simulink model "kf_discrete_time_1_input"  (R2018b)
settings: Solver=FixedStepAuto  StartTime=0.0  StopTime=15  FixedStep=1e-3  RelTol=1e-3
values from neighbouring files (symbols this model uses):
  A = obj.A    [LeftLaneChangeRelativeMotionModel.m]    (also in initialization.m = 1.75; laneChangeSinusoidalFcn.m = 1.75; laneChangeSinusoidalJacobianFcn.m = 1.75; leftLaneChangeParametricFcn.m = lateral_dist/2)
  Ts = 0.1    [KinematicBicycleModel.m]    (also in LeftLaneChangeSinusoidalMotionModel.m; LinearizedBicycleModel.m; SimplifiedKinematicBicycleModel.m; amm_rel_test.m)
  vx = X(2)    [cv_model_fun.m]    (also in initialization.m = 10)
  vy = X(4)    [cv_model_fun.m]    (also in initialization.m = 0)
  w = obj.w    [LeftLaneChangeRelativeMotionModel.m]    (also in ctra_model_fun.m = X(6); ctrv_model_fun.m = X(5); initialization.m = 0.0314159265359; laneChangeSinusoidalFcn.m = 0.0209439510239)
  x = X(1)    [KinematicBicycleModel.m]    (also in SimplifiedKinematicBicycleModel.m; behavior_model.m = 0:0.01:20; cca_model_fun.m; ctra_model_fun.m)
  y = X(2)    [KinematicBicycleModel.m]    (also in SimplifiedKinematicBicycleModel.m; behavior_model.m = [distances velocities]; cca_model_fun.m; ctra_model_fun.m)
  y_init = lanewidth/2    (= 1.75)    [initialization.m]    (also in laneChangeSinusoidalFcn.m; laneChangeSinusoidalJacobianFcn.m; leftLaneChangeSinusoidalFcn.m; leftLaneChangeSinusoidalJacobianFcn.m)
undefined symbols (not defined in the file or in its folder): Discrete, Time
libraries: simulink x8, sharedTrackingLibrary x2, ctrlSharedLib x1
settings Model: Creator=jasprit  LastModifiedBy=jasprit
settings SFSimCC: SimUseLocalCustomCode=off
settings RTWCC: RTWUseLocalCustomCode=off

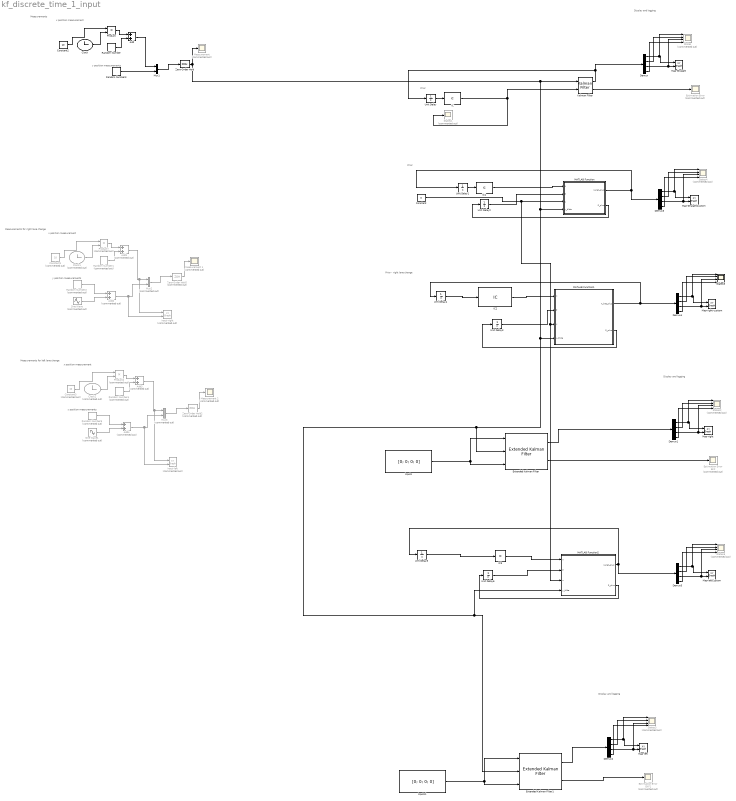
== system kf_discrete_time_1_input ==
  note: Prior - right lane change
  note: Prior
  note: y position measurements
  note: x position measurement
  note: Display and logging
  note: Prior
  note: Measurements
  note: x position measurement
  note: Display and logging
  note: Measurements for right lane change
  note: y position measurements
  note: y position measurements
  note: Measurements for left lane change
  note: Display and logging
  note: x position measurement
  Add : Sum
  Add{1..4} (4 alike) : Sum  Commented=on
  Clock : Clock
  Clock1 : Clock  Commented=on
  Clock2 : Clock  Commented=on
  Constant : Constant  Value=0
  Constant1 : Constant  Commented=on  Value=10
  Constant2 : Constant  Value=10
  Constant3 : Constant  Commented=on  Value=10
  Demux{,1..5} (6 alike) : Demux
  Estimation Error : Scope  Commented=on
  Estimation Error EKF : Scope  Commented=on
  Estimation Error EKF1 : Scope  Commented=on
  Extended Kalman Filter : sharedTrackingLibrary/Extended Kalman Filter  StateTransitionFcn=laneChangeSinusoidalFcn  HasStateTransitionJacobianFcn=on  StateTransitionJacobianFcn=laneChangeSinusoidalJacobianFcn  HasAdditiveProcessNoise=Additive  ProcessNoise=[0.5 5 0.5 5]'  HasTimeVaryingProcessNoise=off  HasStateTransitionFcnExtraArgument=1  InitialState=[x vx y vy]  InitialStateCovariance=1e-6  MeasurementFcn1=positionMeasurementFcn  HasMeasurementJacobianFcn1=off  HasMeasurementEnablePort1=off  HasAdditiveMeasurementNoise1=Additive  MeasurementNoise1=[0.2 0; 0 0.2]  HasTimeVaryingMeasurementNoise1=off  HasMeasurementFcnExtraArgument1=1  MeasurementFcn2=myMeasurementFcn  HasMeasurementJacobianFcn2=off  HasMeasurementEnablePort2=off  HasAdditiveMeasurementNoise2=Additive  MeasurementNoise2=1  HasTimeVaryingMeasurementNoise2=off  HasMeasurementFcnExtraArgument2=0  MeasurementFcn3=myMeasurementFcn  HasMeasurementJacobianFcn3=off  HasMeasurementEnablePort3=off  HasAdditiveMeasurementNoise3=Additive  MeasurementNoise3=1  HasTimeVaryingMeasurementNoise3=off  HasMeasurementFcnExtraArgument3=0  MeasurementFcn4=myMeasurementFcn  HasMeasurementJacobianFcn4=off  HasMeasurementEnablePort4=off  HasAdditiveMeasurementNoise4=Additive  MeasurementNoise4=1  HasTimeVaryingMeasurementNoise4=off  HasMeasurementFcnExtraArgument4=0  MeasurementFcn5=myMeasurementFcn  HasMeasurementJacobianFcn5=off  HasMeasurementEnablePort5=off  HasAdditiveMeasurementNoise5=Additive  MeasurementNoise5=1  HasTimeVaryingMeasurementNoise5=off  HasMeasurementFcnExtraArgument5=0  EnableMultirate=off  StateTransitionFcnSampleTime=1  MeasurementFcn1SampleTime=1  MeasurementFcn2SampleTime=1  MeasurementFcn3SampleTime=1  MeasurementFcn4SampleTime=1  MeasurementFcn5SampleTime=1  UseCurrentEstimator=on  OutputStateCovariance=on  DataType=double  SampleTime=Ts  NumberOfMeasurements=1
      settings: SourceProductName=Control System Toolbox  SourceProductBaseCode=CT
  Extended Kalman Filter1 : sharedTrackingLibrary/Extended Kalman Filter  StateTransitionFcn=leftLaneChangeSinusoidalFcn  HasStateTransitionJacobianFcn=on  StateTransitionJacobianFcn=leftLaneChangeSinusoidalJacobianFcn  HasAdditiveProcessNoise=Additive  ProcessNoise=[0.5 5 0.5 5]'  HasTimeVaryingProcessNoise=off  HasStateTransitionFcnExtraArgument=1  InitialState=[x vx y vy]  InitialStateCovariance=1e-6  MeasurementFcn1=positionMeasurementFcn  HasMeasurementJacobianFcn1=off  HasMeasurementEnablePort1=off  HasAdditiveMeasurementNoise1=Additive  MeasurementNoise1=[0.2 0; 0 0.2]  HasTimeVaryingMeasurementNoise1=off  HasMeasurementFcnExtraArgument1=1  MeasurementFcn2=myMeasurementFcn  HasMeasurementJacobianFcn2=off  HasMeasurementEnablePort2=off  HasAdditiveMeasurementNoise2=Additive  MeasurementNoise2=1  HasTimeVaryingMeasurementNoise2=off  HasMeasurementFcnExtraArgument2=0  MeasurementFcn3=myMeasurementFcn  HasMeasurementJacobianFcn3=off  HasMeasurementEnablePort3=off  HasAdditiveMeasurementNoise3=Additive  MeasurementNoise3=1  HasTimeVaryingMeasurementNoise3=off  HasMeasurementFcnExtraArgument3=0  MeasurementFcn4=myMeasurementFcn  HasMeasurementJacobianFcn4=off  HasMeasurementEnablePort4=off  HasAdditiveMeasurementNoise4=Additive  MeasurementNoise4=1  HasTimeVaryingMeasurementNoise4=off  HasMeasurementFcnExtraArgument4=0  MeasurementFcn5=myMeasurementFcn  HasMeasurementJacobianFcn5=off  HasMeasurementEnablePort5=off  HasAdditiveMeasurementNoise5=Additive  MeasurementNoise5=1  HasTimeVaryingMeasurementNoise5=off  HasMeasurementFcnExtraArgument5=0  EnableMultirate=off  StateTransitionFcnSampleTime=1  MeasurementFcn1SampleTime=1  MeasurementFcn2SampleTime=1  MeasurementFcn3SampleTime=1  MeasurementFcn4SampleTime=1  MeasurementFcn5SampleTime=1  UseCurrentEstimator=on  OutputStateCovariance=on  DataType=double  SampleTime=Ts  NumberOfMeasurements=1
      settings: SourceProductName=Control System Toolbox  SourceProductBaseCode=CT
  IC{,1..3} (4 alike) : InitialCondition  Value=[x vx y vy]
  Inputs : Constant  Value=[0; 0; 0; 0]  SampleTime=Ts
  Inputs1 : Constant  Value=[0; 0; 0; 0]  SampleTime=Ts
  Kalman Filter : ctrlSharedLib/Kalman Filter  TimeDomain=Discrete-Time  UseCurrentEstimator=on  ModelSource=Individual A, B, C, D matrices  ModelSourceVariable=ss(0.95,1,1,0,1)  A=[1 Ts 0 0; 0 1 0 0; 0 0 1 Ts; 0 0 0 1]  B=[1 0; 0 1]  C=[1 0 0 0; 0 0 1 0]  D=[0 0; 0 0]  NumberOfStates=1  NumberOfInputs=1  NumberOfOutputs=1  InitialEstimateSource=Input port  X0=[0 0 20 0]  P0=10  UseK=off  UseGH=off  NumberOfProcessNoiseInputs=1  G=1  TimeInvariantG=on  H=0  TimeInvariantH=on  Q=[0.5 5 0.5 5]'  TimeInvariantQ=on  R=[0.2 0; 0 0.2]  TimeInvariantR=on  N=0  TimeInvariantN=on  AddInputPort=off  AddEnablePort=off  OutputEstimatedY=off  OutputP=on  Ts=Ts
      settings: SourceProductBaseCode=CT
  MATLAB Function : MATLAB Function  TreatAsAtomicUnit=on
  MATLAB Function1 : MATLAB Function  TreatAsAtomicUnit=on
  MATLAB Function2 : MATLAB Function  TreatAsAtomicUnit=on
  Map-Straight : simulink/Sinks/XY Graph  xmin=-1  xmax=200  ymin=-20  ymax=20  st=-1
  Map-StraightCustom : simulink/Sinks/XY Graph  xmin=-1  xmax=200  ymin=-20  ymax=20  st=-1
  Map-left : simulink/Sinks/XY Graph  xmin=-1  xmax=200  ymin=-5  ymax=5  st=-1
  Map-leftCustom : simulink/Sinks/XY Graph  xmin=-1  xmax=200  ymin=-5  ymax=5  st=-1
  Map-right : simulink/Sinks/XY Graph  xmin=-1  xmax=200  ymin=-5  ymax=5  st=-1
  Map-right-custom : simulink/Sinks/XY Graph  xmin=-1  xmax=200  ymin=-5  ymax=5  st=-1
  "Measurement " : Scope  Commented=on
  Measurement 1 : Scope  Commented=on
  Measurement 2 : Scope  Commented=on
  Mux1 : Mux  Inputs=2
  Mux2 : Mux  Commented=on  Inputs=2
  Mux3 : Mux  Commented=on  Inputs=2
  Product : Product
  Product1 : Product  Commented=on
  Product2 : Product  Commented=on
  Random Number : RandomNumber  Variance=0.1  SampleTime=Ts
  Random Number1 : RandomNumber  Commented=on  Variance=0.1  SampleTime=Ts
  Random Number2 : RandomNumber  Commented=on  Variance=0.2  SampleTime=Ts
  Random Number3 : RandomNumber  Variance=0.2  SampleTime=Ts
  Random Number4 : RandomNumber  Commented=on  Variance=0.1  SampleTime=Ts
  Random Number5 : RandomNumber  Commented=on  Variance=0.2  SampleTime=Ts
  Sine Wave : Sin  Commented=on  Amplitude=A  Bias=-A  Frequency=w*vx  Phase=+pi/2  SampleTime=Ts
  Sine Wave1 : Sin  Commented=on  Amplitude=A  Bias=y_init  Frequency=w*vx  Phase=-pi/2  SampleTime=Ts
  States{,2..4,6} (5 alike) : Scope  Commented=on  NumInputPorts=4
  States1 : Scope  Commented=on
  States5 : Scope  NumInputPorts=4
  Unit Delay{,1,4..6} (5 alike) : UnitDelay  SampleTime=-1
  Unit Delay2 : UnitDelay  InitialCondition=1e-6  SampleTime=-1
  Unit Delay3 : UnitDelay  InitialCondition=1e-6  SampleTime=-1
  Zero-Order Hold : ZeroOrderHold  SampleTime=Ts
  Zero-Order Hold1 : ZeroOrderHold  Commented=on  SampleTime=Ts
  Zero-Order Hold2 : ZeroOrderHold  Commented=on  SampleTime=Ts
  input-left : simulink/Sinks/XY Graph  Commented=on  xmin=-1  xmax=200  ymin=-5  ymax=5  st=-1
  input-right : simulink/Sinks/XY Graph  Commented=on  xmin=-1  xmax=200  ymin=-5  ymax=5  st=-1
  wires:
  Constant2/1 -> Product/1
  Kalman Filter/1 -> Demux/1, Unit Delay/1
  Demux/1 -> States/1, Map-Straight/1
  Clock/1 -> Product/2
  Product/1 -> Add/1
  Random Number/1 -> Add/2
  Add/1 -> Mux1/1
  Kalman Filter/2 -> Estimation Error/1
  Demux/2 -> States/2
  Mux1/1 -> Zero-Order Hold/1
  Random Number3/1 -> Mux1/2
  Demux/3 -> Map-Straight/2, States/3
  Demux/4 -> States/4
  IC/1 -> States1/1, Kalman Filter/2
  Unit Delay/1 -> IC/1
  Zero-Order Hold1/1 -> Measurement 1/1
  Extended Kalman Filter/1 -> Demux1/1
  Demux1/4 -> States2/4
  Demux1/1 -> States2/1, Map-right/1
  Product1/1 -> Add1/1
  Clock1/1 -> Product1/2
  Constant1/1 -> Product1/1
  Demux1/2 -> States2/2
  Mux2/1 -> Zero-Order Hold1/1
  Add1/1 -> input-right/1, Mux2/1
  Demux1/3 -> Map-right/2, States2/3
  Random Number1/1 -> Add1/2
  Random Number2/1 -> Add2/1
  Sine Wave/1 -> Add2/2
  Add2/1 -> input-right/2, Mux2/2
  Inputs/1 -> Extended Kalman Filter/3, Extended Kalman Filter/1
  Extended Kalman Filter/2 -> Estimation Error EKF/1
  Random Number5/1 -> Add4/1
  Add3/1 -> input-left/1, Mux3/1
  Clock2/1 -> Product2/2
  Sine Wave1/1 -> Add4/2
  Extended Kalman Filter1/1 -> Demux2/1
  Product2/1 -> Add3/1
  Demux2/2 -> States3/2
  Random Number4/1 -> Add3/2
  Constant3/1 -> Product2/1
  Extended Kalman Filter1/2 -> Estimation Error EKF1/1
  Mux3/1 -> Zero-Order Hold2/1
  Demux2/4 -> States3/4
  Demux2/3 -> Map-left/2, States3/3
  Demux2/1 -> States3/1, Map-left/1
  Add4/1 -> input-left/2, Mux3/2
  Zero-Order Hold2/1 -> Measurement 2/1
  Inputs1/1 -> Extended Kalman Filter1/3, Extended Kalman Filter1/1
  Zero-Order Hold/1 -> MATLAB Function1/4(y_tilde), MATLAB Function2/4(y_tilde), Extended Kalman Filter1/2, Extended Kalman Filter/2, MATLAB Function/4(y_tilde), Kalman Filter/1, "Measurement "/1
  Demux3/1 -> States4/1, Map-StraightCustom/1
  MATLAB Function/1(X_hat_plus) -> Demux3/1, Unit Delay1/1
  Demux3/4 -> States4/4
  Demux3/2 -> States4/2
  Demux3/3 -> Map-StraightCustom/2, States4/3
  IC1/1 -> MATLAB Function/1(X)
  Unit Delay1/1 -> IC1/1
  MATLAB Function/2(P_plus) -> Unit Delay2/1
  Unit Delay2/1 -> MATLAB Function/2(P)
  Constant/1 -> MATLAB Function2/3(u), MATLAB Function1/3(u), MATLAB Function/3(u)
  Demux4/1 -> States5/1, Map-right-custom/1
  Demux4/2 -> States5/2
  MATLAB Function1/1(X_hat_plus) -> Unit Delay4/1, Demux4/1
  Demux4/4 -> States5/4
  Demux4/3 -> Map-right-custom/2, States5/3
  MATLAB Function1/2(P_plus) -> Unit Delay3/1
  Unit Delay3/1 -> MATLAB Function1/2(P)
  IC2/1 -> MATLAB Function1/1(X)
  Unit Delay4/1 -> IC2/1
  IC3/1 -> MATLAB Function2/1(X)
  Unit Delay5/1 -> IC3/1
  MATLAB Function2/2(P_plus) -> Unit Delay6/1
  Unit Delay6/1 -> MATLAB Function2/2(P)
  Demux5/1 -> States6/1, Map-leftCustom/1
  Demux5/4 -> States6/4
  MATLAB Function2/1(X_hat_plus) -> Unit Delay5/1, Demux5/1
  Demux5/3 -> Map-leftCustom/2, States6/3
  Demux5/2 -> States6/2

== matlab function kf_discrete_time_1_input/MATLAB Function1 ==
  data: X input; P input; u input; X_hat_plus output; y_tilde input; P_plus output
function [X_hat_plus, P_plus] = EKFRightLaneChangeCustom(X, P, u, y_tilde)

    %%
    %TODO: See how can this be moved out of the function later
    %sampling time
    Ts = 0.01;

    % measurement noise std deviation (for covariance)
    R = [0.2 0; 0 0.2];
    
    % process noise covariance
    Q = diag([0.5 5.0 0.5 5.0]);

    % states - X = [x vx y vy] -     
    Ck = [1 0 0 0; 0 0 1 0];

    F = laneChangeSinusoidalJacobianFcn(X, u);
    %%
    % Now estimate states using kalman filter
    
    %predict
    xhat_minus = laneChangeSinusoidalFcn(X, u);
    P_minus = (F * P * F') + Ts*Q;
    yhat_minus = Ck * xhat_minus;

    %correct
    covariance_term = Ck * P_minus *Ck';
    inverse_term = inv( covariance_term + R);
    K = P_minus * Ck' * inverse_term;
    X_hat_plus = xhat_minus + K * (y_tilde - yhat_minus);
    P_plus = (eye(4) - K * Ck) * P_minus;
    
    %This will be likely outside
    %e = xhat_plus - x(:, i+1);
    
end

== matlab function kf_discrete_time_1_input/MATLAB Function ==
  data: X input; P input; u input; X_hat_plus output; y_tilde input; P_plus output
function [X_hat_plus, P_plus] = kalmanFilterCustom(X, P, u, y_tilde)

    %%
    %TODO: See how can this be moved out of the function later
    %sampling time
    Ts = 0.01;

    % measurement noise std deviation (for covariance)
    R = [0.2 0; 0 0.2];
    
    % process noise covariance
    Q = diag([0.5 5.0 0.5 5.0]);

    % states - X = [x vx y vy] - 
    
    Ak = [1 Ts 0 0; 0 1 0 0; 0 0 1 Ts; 0 0 0 1];
    Bk = 0;
    Ck = [1 0 0 0; 0 0 1 0];
    Dk = 0;

    %%
    % Now estimate states using kalman filter
    
    %predict
    xhat_minus = Ak * X + Bk * u;
    P_minus = (Ak * P *Ak') + Ts*Q;
    yhat_minus = Ck * xhat_minus;

    %correct
    covariance_term = Ck * P_minus *Ck';
    inverse_term = inv( covariance_term + R);
    K = P_minus * Ck' * inverse_term;
    X_hat_plus = xhat_minus + K * (y_tilde - yhat_minus);
    P_plus = (eye(4) - K * Ck) * P_minus;
    
    %This will be likely outside
    %e = xhat_plus - x(:, i+1);
    
end

== matlab function kf_discrete_time_1_input/MATLAB Function2 ==
  data: X input; P input; u input; X_hat_plus output; y_tilde input; P_plus output
function [X_hat_plus, P_plus] = EKFLeftLaneChangeCustom(X, P, u, y_tilde)

    %%
    %TODO: See how can this be moved out of the function later
    %sampling time
    Ts = 0.01;

    % measurement noise std deviation (for covariance)
    R = [0.2 0; 0 0.2];
    
    % process noise covariance
    Q = diag([0.5 5.0 0.5 5.0]);

    % states - X = [x vx y vy] -     
    Ck = [1 0 0 0; 0 0 1 0];

    F = leftLaneChangeSinusoidalJacobianFcn(X, u);
    %%
    % Now estimate states using kalman filter
    
    %predict
    xhat_minus = leftLaneChangeSinusoidalFcn(X, u);
    P_minus = (F * P * F') + Ts*Q;
    yhat_minus = Ck * xhat_minus;

    %correct
    covariance_term = Ck * P_minus *Ck';
    inverse_term = inv( covariance_term + R);
    K = P_minus * Ck' * inverse_term;
    X_hat_plus = xhat_minus + K * (y_tilde - yhat_minus);
    P_plus = (eye(4) - K * Ck) * P_minus;
    
    %This will be likely outside
    %e = xhat_plus - x(:, i+1);
    
end
